simulink model "Scheduler"  (R2020b)
settings: Solver=FixedStepAuto  StartTime=0.0  StopTime=Inf  FixedStep=SAMPLING_TIME  RelTol=1e-3
undefined symbols (not defined in the file): SAMPLING_TIME
libraries: Components x7
Description:
  | % Copyright 2019 The MathWorks, Inc.
settings Model: DataDictionary=Parameters.sldd  EnableAccessToBaseWorkspace=off  EnablePacing=on  Creator=sdupertu  LastModifiedBy=sebas
settings DataIOCC: SaveOutput=off  SaveTime=off
settings OptimizationCC: DefaultParameterBehavior=Inlined  EnhancedBackFolding=on  PassReuseOutputArgsAs=Individual arguments  OptimizeBlockOrder=speed  DifferentSizesBufferReuse=on  OptimizationCustomize=off  EfficientTunableParamExpr=on
settings DebuggingCC: ParameterTunabilityLossMsg=error  PregeneratedLibrarySubsystemCodeDiagnostic=none  ArithmeticOperatorsInVariantConditions=warning
settings ModelReferenceCC: EnableParallelModelReferenceBuilds=on
settings SFSimCC: SimUseLocalCustomCode=off  MATLABDynamicMemAlloc=off  CustomCodeUndefinedFunction=UseInterfaceOnly
settings RTWCC: Description=Embedded Coder  SystemTargetFile=ert.tlc  TemplateMakefile=ert_default_tmf  GenerateReport=on  RTWUseLocalCustomCode=off  IncludeHyperlinkInReport=on  LaunchReport=on  GenerateTraceInfo=on  GenerateTraceReport=on  GenerateTraceReportSl=on  GenerateTraceReportSf=on  GenerateTraceReportEml=on  GenerateWebview=on  GenerateCodeMetricsReport=on
settings CodeAppCC: ForceParamTrailComments=on  IgnoreCustomStorageClasses=off  MaxIdLength=61  OperatorAnnotations=on  SimulinkDataObjDesc=on  SFDataObjDesc=on  InsertBlockDesc=on
settings ERTTargetCC: TargetLangStandard=C99 (ISO)  GenerateSampleERTMain=on  CombineOutputUpdateFcns=off  InlinedParameterPlacement=NonHierarchical  ERTCustomFileTemplate=example_file_process.tlc

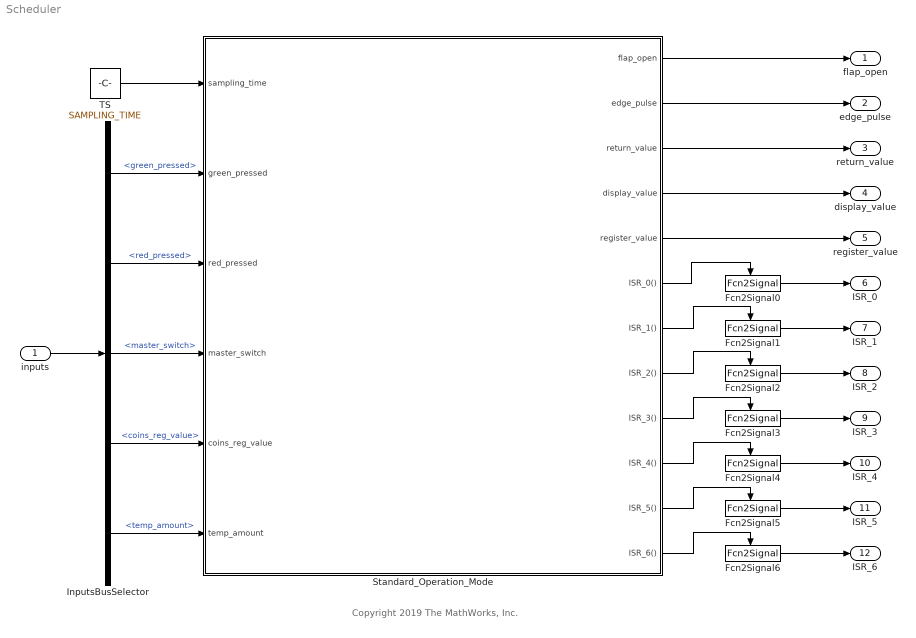
== system Scheduler ==
  note: Copyright 2019 The MathWorks, Inc.
  inputs : Inport  OutDataTypeStr=Bus: InputsBus
  Fcn2Signal{0..6} (7 alike) : Components/Fcn2Signal  SystemSampleTime=-1  VariantActivationTime=update diagram  Latency=0  AutoFrameSizeCalculation=off
  InputsBusSelector : BusSelector  OutputSignals=green_pressed,red_pressed,master_switch,coins_reg_value,temp_amount
  Standard_Operation_Mode : Stateflow chart  TreatAsAtomicUnit=on
  TS : Constant  Value=SAMPLING_TIME  SampleTime=-1
  flap_open : Outport  OutDataTypeStr=boolean  VectorParamsAs1DForOutWhenUnconnected=off
  edge_pulse : Outport  Port=2  OutDataTypeStr=boolean  VectorParamsAs1DForOutWhenUnconnected=off
  return_value : Outport  Port=3  OutDataTypeStr=uint8  VectorParamsAs1DForOutWhenUnconnected=off
  display_value : Outport  Port=4  OutDataTypeStr=uint8  PortDimensions=[1 3]  VectorParamsAs1DForOutWhenUnconnected=off
  register_value : Outport  Port=5  OutDataTypeStr=uint8  VectorParamsAs1DForOutWhenUnconnected=off
  ISR_0 : Outport  Port=6  VectorParamsAs1DForOutWhenUnconnected=off
  ISR_1 : Outport  Port=7  VectorParamsAs1DForOutWhenUnconnected=off
  ISR_2 : Outport  Port=8  VectorParamsAs1DForOutWhenUnconnected=off
  ISR_3 : Outport  Port=9  VectorParamsAs1DForOutWhenUnconnected=off
  ISR_4 : Outport  Port=10  VectorParamsAs1DForOutWhenUnconnected=off
  ISR_5 : Outport  Port=11  VectorParamsAs1DForOutWhenUnconnected=off
  ISR_6 : Outport  Port=12  VectorParamsAs1DForOutWhenUnconnected=off
  wires:
  TS/1 -> Standard_Operation_Mode/1(sampling_time)
  Standard_Operation_Mode/1(flap_open) -> flap_open/1
  Standard_Operation_Mode/2(edge_pulse) -> edge_pulse/1
  Standard_Operation_Mode/4(display_value) -> display_value/1
  Standard_Operation_Mode/3(return_value) -> return_value/1
  Standard_Operation_Mode/5(register_value) -> register_value/1
  Standard_Operation_Mode/6(ISR_0()) -> Fcn2Signal0/Trigger
  Standard_Operation_Mode/7(ISR_1()) -> Fcn2Signal1/Trigger
  Standard_Operation_Mode/8(ISR_2()) -> Fcn2Signal2/Trigger
  Standard_Operation_Mode/9(ISR_3()) -> Fcn2Signal3/Trigger
  Standard_Operation_Mode/10(ISR_4()) -> Fcn2Signal4/Trigger
  Standard_Operation_Mode/11(ISR_5()) -> Fcn2Signal5/Trigger
  Standard_Operation_Mode/12(ISR_6()) -> Fcn2Signal6/Trigger
  Fcn2Signal6/1 -> ISR_6/1
  Fcn2Signal1/1 -> ISR_1/1
  Fcn2Signal2/1 -> ISR_2/1
  Fcn2Signal3/1 -> ISR_3/1
  Fcn2Signal4/1 -> ISR_4/1
  Fcn2Signal5/1 -> ISR_5/1
  Fcn2Signal0/1 -> ISR_0/1
  inputs/1 -> InputsBusSelector/1
  InputsBusSelector/2 -> Standard_Operation_Mode/3(red_pressed)  "<red_pressed>"
  InputsBusSelector/4 -> Standard_Operation_Mode/5(coins_reg_value)  "<coins_reg_value>"
  InputsBusSelector/5 -> Standard_Operation_Mode/6(temp_amount)  "<temp_amount>"
  InputsBusSelector/3 -> Standard_Operation_Mode/4(master_switch)  "<master_switch>"
  InputsBusSelector/1 -> Standard_Operation_Mode/2(green_pressed)  "<green_pressed>"

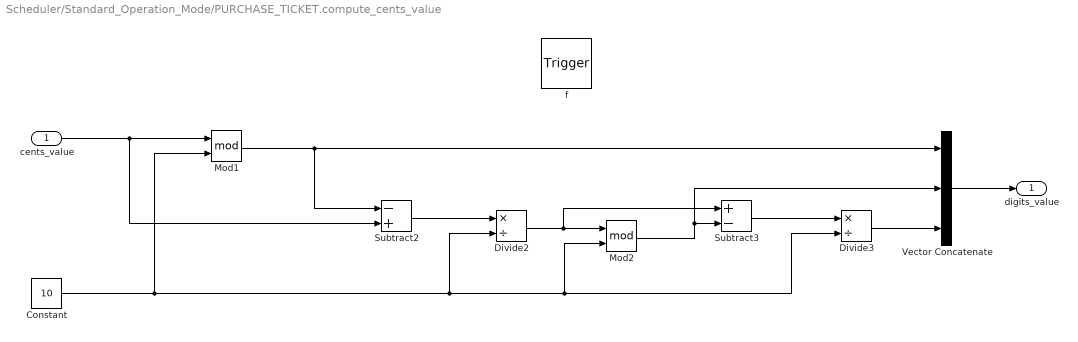
== system Scheduler/Standard_Operation_Mode/PURCHASE_TICKET.compute_cents_value ==
  cents_value : Inport  OutDataTypeStr=uint8  PortDimensions=[1 1]
  f : TriggerPort  TriggerType=function-call  VariantControl=(inherit)
      settings: CopyFcn=Stateflow.SLINSF.SimulinkMan.removeBlockPreDeleteFcn  PreDeleteFcn=Stateflow.SLINSF.SimulinkMan.unsafePredeleteFcn
  Constant : Constant  Value=10  OutDataTypeStr=uint8
  Divide2 : Product  Inputs=*/
  Divide3 : Product  Inputs=*/
  Mod1 : Math  Operator=mod  SignedPower=on  SaturateOnIntegerOverflow=on
  Mod2 : Math  Operator=mod  SignedPower=on  SaturateOnIntegerOverflow=on
  Subtract2 : Sum  Inputs=-+
  Subtract3 : Sum  Inputs=+-
  Vector Concatenate : Concatenate  NumInputs=3
  digits_value : Outport  PortDimensions=[1 3]  VectorParamsAs1DForOutWhenUnconnected=off
  wires:
  cents_value/1 -> Mod1/1, Subtract2/2
  Mod1/1 -> Subtract2/1, Vector Concatenate/1
  Vector Concatenate/1 -> digits_value/1
  Subtract2/1 -> Divide2/1
  Divide2/1 -> Subtract3/1, Mod2/1
  Mod2/1 -> Subtract3/2, Vector Concatenate/2
  Divide3/1 -> Vector Concatenate/3
  Constant/1 -> Mod2/2, Divide3/2, Divide2/2, Mod1/2
  Subtract3/1 -> Divide3/1

== stateflow chart Scheduler/Standard_Operation_Mode ==
  state INITIALIZATION
    during: % Reset of the parking meter status
    display_value = uint8(double(SEGMENTS_DIGIT_M)*ones(1,NB_DISP));
    flap_open = logical(0);
    send(ISR_1); % Initial state of the 7 segments displays
    send(ISR_2); % Close the coin's flap
    send(ISR_5); % Check the status of the green button and master switch
  state PURCHASE_CHECK
    entry: % Waiting on a ticket purchase request
    send(ISR_3); % Ignit the checking of the money that can be given back
    send(ISR_5); % Ignit the checking of the green button and master switch
    during:
    send(ISR_3); % Leds: check if the parking meter can give money back
    send(ISR_5); % Check the status of the green button and master switch
  state STOP_EXECUTION
    during: % Stop the model execution
    send(ISR_0); % Trigger the terminate function to stop the execution
  state CHECK_COINS
    entry: % Update of the button value state once it has been pressed
    send(ISR_5); % Status of the green button must be equal to zero
    during:
    display_value = [SEGMENTS_DIGIT_0, SEGMENTS_DIGIT_2, ...
    SEGMENTS_DIGIT_1+SEGMENTS_DIGIT_P];
    flap_open = logical(1);
    % Send interrupts
    send(ISR_1); % Display the cost of a parking ticket
    send(ISR_2); % Open the coin's flap
  state PURCHASE_TICKET
    % Waiting for the full paiment or the cancellation of the ticket
    state digits_value = compute_cents_value(cents_value) [function]
    state INITIALIZATION
      during: % Reset local variables and pause the process
      inserted_amount = uint16(0);
      amount_to_return = uint8(0);
      register_value = uint8(0);
      remaining_amount = uint8(zeros(1,3));
    state CANCEL_CHECK
      during: % Check if the purchase is being cancelled
      send(ISR_5); % Check status of the red button
    state CANCEL_PURCHASE
      during: % Ticket's purchase process cancelled
      amount_to_return = uint8(inserted_amount);
    state COIN_CHECK
      during: % Update the amount to pay if a coin has been inserted
      send(ISR_6); % Check current inserted coin
      inserted_amount = inserted_amount + uint16(temp_amount);
    state COINS_RISING_EDGE
      entry: % Update the amount to pay if a coin has been inserted
      [amount_to_return, return_value] = ...
      return_coins_value(int32(amount_to_return));
      exit:
      edge_pulse = logical(1);
      send(ISR_4); % Rising Edge of the pulse for the coins to give back
    state UPDATE_AMOUNT
      during: % Update the amount to pay if a coin has been inserted
      register_value = coins_reg_value;
      remaining_amount = ...
      compute_cents_value(uint8(TICKET_FEE-inserted_amount));
      display_value = display_digits(remaining_amount);
      display_value(end) = display_value(end)+SEGMENTS_DIGIT_P;
      send(ISR_1); % Update the remaining cents amount to pay
    state COINS_FALLING_EDGE
      exit: % Generate peripherals pulse
      edge_pulse = logical(0);
      send(ISR_4); % Falling Edge of the pulse for the coins to give back
    state COINS_REMAINING
      during: % Remaining coins to give back
    state TICKET_PAID
      during: % Printing of the parking ticket
      display_value = [SEGMENTS_DIGIT_0, SEGMENTS_DIGIT_0, ...
      SEGMENTS_DIGIT_0+SEGMENTS_DIGIT_P];
      send(ISR_1); % Total ticket amount paid
    state RECEIPT_RISING_EDGE
      exit: % Generate peripherals pulse
      edge_pulse = logical(1);
      return_value = INT_MASK_PRINT_TICKET;
      send(ISR_4); % Rising Edge of the pulse for the receipt
    state RECEIPT_FALLING_EDGE
      exit: % Generate peripherals pulse
      edge_pulse = logical(0);
      send(ISR_4); % Falling Edge of the pulse for the receipt
    state GIVE_BACK_CHANGE
      entry: % Give back coin's change
      amount_to_return = uint8(inserted_amount-TICKET_FEE);
    (default) -> PURCHASE_TICKET.INITIALIZATION
    PURCHASE_TICKET.INITIALIZATION -> CANCEL_CHECK : [after(REFRESHING_TICK, tick)]
    CANCEL_CHECK -> CANCEL_PURCHASE [order 1] : [red_pressed == true]
    (junction 96) -> CANCEL_CHECK
    (junction 97) -> (junction 96) : [after(REFRESHING_TICK, tick)]
    CANCEL_PURCHASE -> COINS_RISING_EDGE : [after(REFRESHING_TICK, tick)]
    COIN_CHECK -> CANCEL_CHECK [order 2] : [after(REFRESHING_TICK, tick)]
    CANCEL_CHECK -> COIN_CHECK [order 2] : [after(REFRESHING_TICK, tick)]
    (junction 153) -> COINS_RISING_EDGE
    COIN_CHECK -> UPDATE_AMOUNT [order 1] : [coins_reg_value ~= register_value]
    (junction 154) -> (junction 153) : [amount_to_return > 0]
    COINS_RISING_EDGE -> COINS_FALLING_EDGE : [after(PULSE_DUR_TICK, tick)]
    UPDATE_AMOUNT -> (junction 97) [order 1]
    COINS_FALLING_EDGE -> COINS_REMAINING : [after(PULSE_DUR_TICK, tick)]
    UPDATE_AMOUNT -> TICKET_PAID [order 2] : [inserted_amount >= TICKET_FEE]
    COINS_REMAINING -> (junction 154) [order 1]
    GIVE_BACK_CHANGE -> COINS_REMAINING : [true]
    TICKET_PAID -> RECEIPT_RISING_EDGE : [after(REFRESHING_TICK, tick)]
    RECEIPT_RISING_EDGE -> RECEIPT_FALLING_EDGE : [after(PULSE_DUR_TICK, tick)]
    RECEIPT_FALLING_EDGE -> GIVE_BACK_CHANGE : [after(PULSE_DUR_TICK, tick)]
  (default) -> INITIALIZATION : {REFRESHING_TICK = REFRESHING_TIME/sampling_time;
      |  PULSE_DUR_TICK   = PULSE_DURATION/sampling_time;}
  (junction 59) -> INITIALIZATION
  (junction 58) -> (junction 59)
  INITIALIZATION -> PURCHASE_CHECK : [after(REFRESHING_TICK, tick)]
  PURCHASE_CHECK -> (junction 164) [order 2] : [master_switch == false]
  (junction 164) -> STOP_EXECUTION
  PURCHASE_CHECK -> CHECK_COINS [order 1] : [green_pressed == true]
  CHECK_COINS -> PURCHASE_TICKET : [after(REFRESHING_TICK, tick)]
  COINS_REMAINING -> (junction 58) [order 2]
  data: cents_value function_input uint8 size=[1 1]; digits_value function_output size=[1 3]; new_reg_value function_output; digit_value function_input; amount_back function_output; new_reg_value function_output; amount function_input; sampling_time input; flap_open output boolean =false; edge_pulse output boolean =false; return_value output; display_value output uint8 size=[1 3]; SEGMENTS_DIGIT_M data_store_memory; SEGMENTS_DIGIT_1 data_store_memory; green_pressed input boolean size=[1 1]; SEGMENTS_DIGIT_0 data_store_memory; SEGMENTS_DIGIT_2 data_store_memory; SEGMENTS_DIGIT_P data_store_memory; REFRESHING_TIME data_store_memory; TICKET_FEE data_store_memory; red_pressed input boolean size=[1 1]; master_switch input boolean size=[1 1]; coins_reg_value input; NB_DISP constant uint8 =uint8(3); temp_amount input; remaining_amount local; SEGMENTS_DIGIT_3 data_store_memory; SEGMENTS_DIGIT_4 data_store_memory; SEGMENTS_DIGIT_5 data_store_memory; SEGMENTS_DIGIT_6 data_store_memory; SEGMENTS_DIGIT_7 data_store_memory; SEGMENTS_DIGIT_8 data_store_memory; SEGMENTS_DIGIT_9 data_store_memory; SEGMENTS_DIGIT_E data_store_memory; INT_CASE_ENTRY_0 data_store_memory; INT_CASE_ENTRY_1 data_store_memory; INT_CASE_ENTRY_2 data_store_memory; INT_CASE_ENTRY_3 data_store_memory; INT_CASE_ENTRY_4 data_store_memory; INT_CASE_ENTRY_5 data_store_memory; INT_CASE_ENTRY_6 data_store_memory; INT_CASE_ENTRY_7 data_store_memory; INT_CASE_ENTRY_8 data_store_memory; INT_CASE_ENTRY_9 data_store_memory; INT_CASE_ENTRY_M data_store_memory; inserted_amount local uint16; register_value output; PULSE_DURATION data_store_memory; amount_to_return local; INT_VAL_010_CENTS data_store_memory; INT_VAL_020_CENTS data_store_memory; INT_VAL_050_CENTS data_store_memory; INT_VAL_100_CENTS data_store_memory; INT_MASK_100_CENTS data_store_memory; INT_MASK_010_CENTS data_store_memory; INT_MASK_020_CENTS data_store_memory; INT_MASK_050_CENTS data_store_memory; INT_MASK_PRINT_TICKET data_store_memory; REFRESHING_TICK local; PULSE_DUR_TICK local
  events: ISR_0 output FUNCTION_CALL_EVENT; ISR_1 output FUNCTION_CALL_EVENT; ISR_2 output FUNCTION_CALL_EVENT; ISR_3 output FUNCTION_CALL_EVENT; ISR_4 output FUNCTION_CALL_EVENT; ISR_5 output FUNCTION_CALL_EVENT; ISR_6 output FUNCTION_CALL_EVENT
  function new_reg_value = display_digits(digit_value):
    | function new_reg_value = display_digits(digit_value)
    | %%%%%%%%%%%%%%%%%%%%%%%%%%%%%%%%%%%%%%%%%%%%%%%%%%%%%%%%%%%%%%%%%%%%%%%%%%%%%%%%
    | % Function display_digits()
    | % Goal  : Update the 7 segments displays with new digits values
    | % IN    : - digit_value: base 10 value to display on the 7 segments displays
    | % IN/OUT: -
    | % OUT   : - new_reg_value: array of integers representing the updated amount of
    | %           inserted coins
    | %%%%%%%%%%%%%%%%%%%%%%%%%%%%%%%%%%%%%%%%%%%%%%%%%%%%%%%%%%%%%%%%%%%%%%%%%%%%%%%%
    | %#codegen
    |   new_reg_value = uint8(double(SEGMENTS_DIGIT_E)*ones(1,NB_DISP));
    | 
    |   for i=1:1:NB_DISP
    |     switch (digit_value(i))
    |       case INT_CASE_ENTRY_0
    |         new_reg_value(i) = SEGMENTS_DIGIT_0;
    |       case INT_CASE_ENTRY_1
    |         new_reg_value(i) = SEGMENTS_DIGIT_1;
    |       case INT_CASE_ENTRY_2
    |         new_reg_value(i) = SEGMENTS_DIGIT_2;
    |       case INT_CASE_ENTRY_3
    |         new_reg_value(i) = SEGMENTS_DIGIT_3;
    |       case INT_CASE_ENTRY_4
    |         new_reg_value(i) = SEGMENTS_DIGIT_4;
    |       case INT_CASE_ENTRY_5
    |         new_reg_value(i) = SEGMENTS_DIGIT_5;
    |       case INT_CASE_ENTRY_6
    |         new_reg_value(i) = SEGMENTS_DIGIT_6;
    |       case INT_CASE_ENTRY_7
    |         new_reg_value(i) = SEGMENTS_DIGIT_7;
    |       case INT_CASE_ENTRY_8
    |         new_reg_value(i) = SEGMENTS_DIGIT_8;
    |       case INT_CASE_ENTRY_9
    |         new_reg_value(i) = SEGMENTS_DIGIT_9;
    |       case INT_CASE_ENTRY_M
    |         new_reg_value(i) = SEGMENTS_DIGIT_M;
    |       otherwise
    |         % Incorrect 7 segments encoded value given to the selected HW register
    |         new_reg_value(i) = SEGMENTS_DIGIT_E;
    |     end
    |   end
    | end
  function [amount_back, new_reg_value] = return_coins_value(amount):
    | function [amount_back, new_reg_value] = return_coins_value(amount)
    | %%%%%%%%%%%%%%%%%%%%%%%%%%%%%%%%%%%%%%%%%%%%%%%%%%%%%%%%%%%%%%%%%%%%%%%%%%%%%%%%
    | % Function return_coins_value()
    | % Goal  : 
    | % IN    : - amount: amount corresponding to the coin value to return
    | % IN/OUT: -
    | % OUT   : - new_reg_value: value representing the coin's value to return
    | %%%%%%%%%%%%%%%%%%%%%%%%%%%%%%%%%%%%%%%%%%%%%%%%%%%%%%%%%%%%%%%%%%%%%%%%%%%%%%%%
    | %#codegen
    |   new_reg_value = uint8(0);
    |   amount_back   = uint8(0);
    | 
    |   if (amount - INT_VAL_100_CENTS >= 0)
    |     new_reg_value = INT_MASK_100_CENTS;
    |     amount_back = uint8(amount - INT_VAL_100_CENTS);
    |   elseif (amount - INT_VAL_050_CENTS >= 0)
    |     new_reg_value = INT_MASK_050_CENTS;
    |     amount_back = uint8(amount - INT_VAL_050_CENTS);
    |   elseif (amount - INT_VAL_020_CENTS >= 0)
    |     new_reg_value = INT_MASK_020_CENTS;
    |     amount_back = uint8(amount - INT_VAL_020_CENTS);
    |   elseif (amount - INT_VAL_010_CENTS >= 0)
    |     new_reg_value = INT_MASK_010_CENTS;
    |     amount_back = uint8(amount - INT_VAL_010_CENTS);
    |   end
    | end
